simulink library "Project1_Library"  (R2017b)
settings: Solver=VariableStepAuto  StartTime=0.0  StopTime=10.0  RelTol=1e-3
settings Model: Creator=hattanbadyah  LastModifiedBy=hattanbadyah

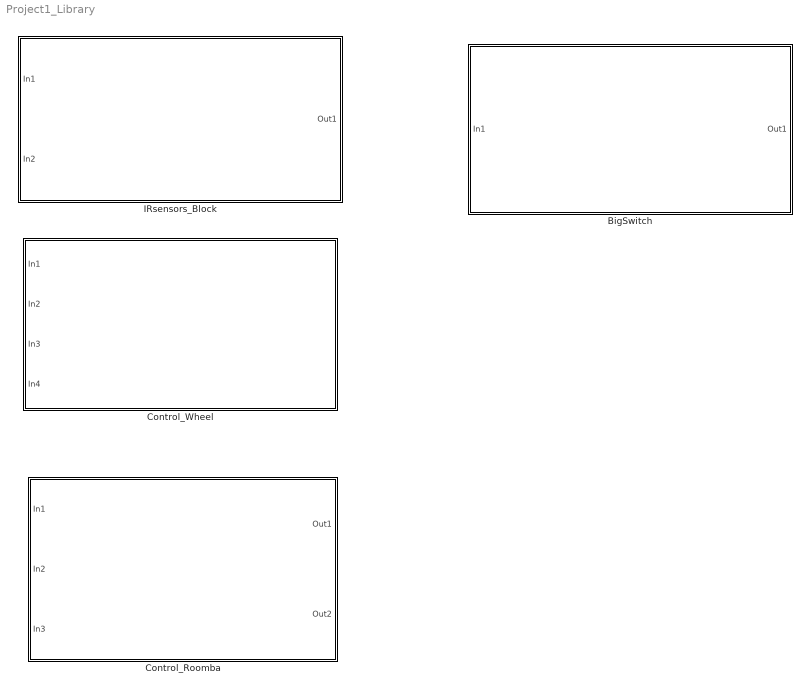
== system Project1_Library ==
  BigSwitch : Subsystem
      mask Help: Click on this link for more information:
      mask Display:
      | disp('BigSwitch');
      | port_label('output',1,'BigSwitch');
      | port_label('input', 1,'manual_switch');
  Control_Roomba : Subsystem
      mask help: This block contains the algorithm to control the Roomba and make it autonomus
      mask Display:
      | disp('Control_Roomba');
      | port_label('input', 1,'SonarSensor');
      | port_label('input', 2,'SonarRanges');
      | port_label('input', 3,'BigSwitch');
      | port_label('output',1,'LeftVel');
      | port_label('output',2,'RightVel');
  Control_Wheel : Subsystem
      mask Help: Click on this link for more information:
      mask Display:
      | disp('Control_Wheel');
      | port_label('input', 1,'LeftW');
      | port_label('input', 2,'RightW');
      | port_label('input', 3,'TurnWheel');
      | port_label('input', 4,'BigSwitch');
  IRsensors_Block : Subsystem
      mask Help: Click on this link for more information
      mask Display:
      | disp('IRsensors_Block');
      | port_label('input',1,'ReadSensor');
      | port_label('input', 2,'BigSwitch');
      | port_label('output', 1,'SensorsRead');

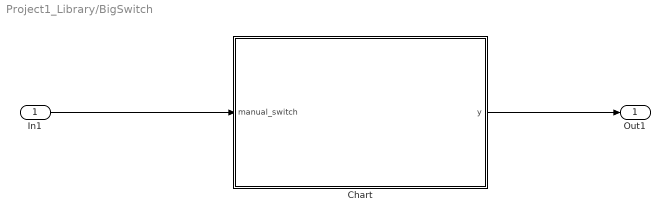
== system Project1_Library/BigSwitch ==
  In1 : Inport
  Chart : Stateflow chart  TreatAsAtomicUnit=on
  Out1 : Outport
  wires:
  In1/1 -> Chart/1(manual_switch)
  Chart/1(y) -> Out1/1

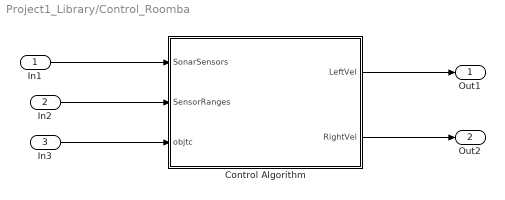
== system Project1_Library/Control_Roomba ==
  In1 : Inport
  In2 : Inport  Port=2
  In3 : Inport  Port=3
  Control Algorithm : Stateflow chart  TreatAsAtomicUnit=on  mask{v0=0.05}
      mask prompts: v0 "Wheel Angular Velocity"
  Out1 : Outport
  Out2 : Outport  Port=2
  wires:
  In1/1 -> Control Algorithm/1(SonarSensors)
  In2/1 -> Control Algorithm/2(SensorRanges)
  In3/1 -> Control Algorithm/3(objtc)
  Control Algorithm/1(LeftVel) -> Out1/1
  Control Algorithm/2(RightVel) -> Out2/1

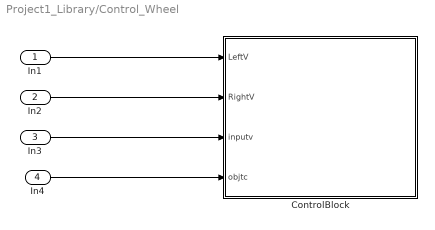
== system Project1_Library/Control_Wheel ==
  In1 : Inport
  In2 : Inport  Port=2
  In3 : Inport  Port=3
  In4 : Inport  Port=4
  ControlBlock : Stateflow chart  TreatAsAtomicUnit=on
  wires:
  In1/1 -> ControlBlock/1(LeftV)
  In2/1 -> ControlBlock/2(RightV)
  In3/1 -> ControlBlock/3(inputv)
  In4/1 -> ControlBlock/4(objtc)

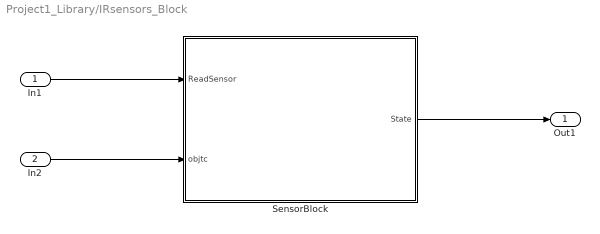
== system Project1_Library/IRsensors_Block ==
  In1 : Inport
  In2 : Inport  Port=2
  SensorBlock : Stateflow chart  TreatAsAtomicUnit=on
  Out1 : Outport
  wires:
  In1/1 -> SensorBlock/1(ReadSensor)
  In2/1 -> SensorBlock/2(objtc)
  SensorBlock/1(State) -> Out1/1

== stateflow chart Project1_Library/IRsensors_Block/SensorBlock ==
  state A
  state Start
    entry, during:
    coder.extrinsic('evalin')
    so=evalin('base','objWs');
    %status = 0
  state Sensor
    entry, during:
    coder.extrinsic('RangeStateRoomba');
    State=RangeStateRoomba(so);
    %status = 1;
  (default) -> A
  A -> Start : [objtc==1]
  Start -> Sensor : [ReadSensor==1]
  Sensor -> Start : [ReadSensor==0]
  data: ReadSensor input; so local; State output double size=6; objtc input

== stateflow chart Project1_Library/BigSwitch/Chart ==
  state A
    en,du:
    tcpInit;
  state Connect
    entry:
    y=1
  state Disconnect
    entry: coder.extrinsic('evalin');
    so=evalin('base','objWs');
    fclose(so);
  state Refresh1
    entry:
    y = y + 1
    if y==4
    y = 1
    end
  state Refresh
    entry:
    y = y + 1
  (default) -> A
  Disconnect -> A : [manual_switch==1]
  A -> Connect : [manual_switch==1]
  Refresh1 -> Connect [order 1] : [manual_switch==1]
  Connect -> Refresh : [manual_switch==1]
  Refresh1 -> Disconnect [order 2] : [manual_switch==0]
  Refresh -> Refresh1 : [manual_switch==1 ]
  data: manual_switch input; so local; y output
  function tcpInit:
    | function tcpInit
    | coder.extrinsic('tcpip');
    | coder.extrinsic('assignin');
    | persistent obj
    | if isempty(obj)
    |     obj=tcpip('10.0.0.1',9001);
    |     set(obj,'Terminator','LF')
    |     set(obj,'InputBufferSize',1000)
    |     set(obj, 'Timeout', 1)
    |     set(obj, 'ByteOrder','bigEndian');
    |     assignin('base','objWs',obj);
    |     
    | fopen(obj);
    |     % Start!
    | Start=[128];
    | fwrite(obj,Start);
    | pause(.1)
    | Mode=[132]
    | fwrite(obj,Mode);
    | pause(.1)
    | 
    | % %Print 'go' on display
    | fwrite(obj, [164, 71, 79, 32, 32]);
    | % make a sound
    | fwrite(obj, [140 1 3 60 20 72 20 84 40 ]); %RoombaInit Song
    | fwrite(obj, [140 2 1 60 20]); % BeepRoomba song
    | fwrite(obj, [140 3 3 84 20 72 30 60 40]); % PowerOffRoomba song
    | fwrite(obj, [141 1]); % play RoombaInit song
    | disp('Robot should display go on 7 segment LED panel and play song.')
    | pause(1);
    | end

== stateflow chart Project1_Library/Control_Wheel/ControlBlock ==
  state blank
  state Connect
    entry:
    coder.extrinsic('evalin');
    obj=evalin('base','objWs');
    %status= 0
  state Reset_Stop
    entry:
    coder.extrinsic('SetWheelVelRoomba')
    SetWheelVelRoomba(obj,0, 0)
    %status=2
  state Update
    entry,during:
    coder.extrinsic('SetWheelVelRoomba')
    SetWheelVelRoomba(obj,RightV, LeftV)
    %status=1
  state start
    entry,during:
    coder.extrinsic('SetWheelVelRoomba')
    SetWheelVelRoomba(obj,RightV, LeftV)
    %status=1
  (default) -> blank
  blank -> Connect : [objtc==2]
  Reset_Stop -> Connect [order 2] : after(30,sec)
  Connect -> start : [inputv==1]
  Update -> start : after(0.5,sec)
  start -> Reset_Stop [order 1] : [inputv==0]
  Reset_Stop -> start [order 1] : [inputv==1]
  start -> Update [order 2] : after(0.5,sec)
  data: LeftV input; RightV input; inputv input; objtc input; obj local

== stateflow chart Project1_Library/Control_Roomba/Control Algorithm ==
  state Begin
  state Control_Roomba
    en,du:
    coder.extrinsic('evalin');
    so=evalin('base','objWs');
    coder.extrinsic('PowerOffRoomba');
    coder.extrinsic('BatteryChargeReaderRoomba');
    coder.extrinsic('BeepRoomba');
    coder.extrinsic('BumpsWheelDropsSensorsRoomba');
    b_s= BumpsWheelDropsSensorsRoomba(so);
    coder.extrinsic('SeekDockRoomba');
    state Controling_Logic [parallel]
      en,du:
      RHS = [SonarSensors(4:6)] > SensorRanges(4:6);
      LHS = [SonarSensors(1:3)] > SensorRanges(1:3);
      MRS = [SonarSensors(5:6)] > SensorRanges(5:6);
      FRS = [SonarSensors(4:5)] > SensorRanges(4:5);
      FMS = [SonarSensors(3:4) ]> SensorRanges(3:4);
      FLS=[SonarSensors(2:3)]>SensorRanges(2:3);
      MLS=[SonarSensors(1:2)]>SensorRanges(1:2);
      RS1=[SonarSensors(6)]>SensorRanges(6);
      RS2=[SonarSensors(5)]>SensorRanges(5);
      RS3=[SonarSensors(4)]>SensorRanges(4);
      LS3=[SonarSensors(3)]>SensorRanges(3);
      LS2=[SonarSensors(2)]>SensorRanges(2);
      LS1=[SonarSensors(1)]>SensorRanges(1);
      R_bump=0;
      R_bump=b_s(1);
      L_bump=0;
      L_bump=b_s(2);
      F_bump=0;
      F_bump=b_s(3);
      WD_R=0;
      WD_R=b_s(4);
      WD_L=0;
      WD_L=b_s(5) ;
      settings: executionOrder=2
      state Start
      state Choose_None3
        en,du:
        RightVel=-v0;
        LeftVel=v0;
      state test_bump
        en,du:
        RightVel=-v0;
        LeftVel=-v0;
      state Choose_None
        en,du:
        RightVel= v0
        LeftVel= v0
      state Choose_None1
        en,du:
        RightVel= -v0
        LeftVel= v0
      state Front_S
        en,du:
        RightVel= -v0
        LeftVel= -v0
      state Choose_State
      state Choose_Between1
      state Choose_Between
      state Pick_LHS
        en,du:
        RightVel= -v0;
        LeftVel= -v0;
      state Pick_RHS
        en,du:
        RightVel= -v0;
        LeftVel= -v0;
      state Pick_RS3
        en,du:
        RightVel= v0;
        LeftVel= -v0 ;
      state Pick_RS2
        en,du:
        RightVel= v0;
        LeftVel= -v0;
      state Pick_MRS
        en,du:
        RightVel= v0;
        LeftVel= -v0;
      state Pick_FRS
        en,du:
        RightVel= v0;
        LeftVel= -v0;
      state Pick_RS1
        en,du:
        RightVel= v0;
        LeftVel= -v0;
      state Pick_LS3
        en,du:
        RightVel= -v0;
        LeftVel= v0;
      state Pick_MLS
        en,du:
        RightVel= -v0;
        LeftVel= v0;
      state Pick_FLS
        en,du:
        RightVel= -v0;
        LeftVel= v0;
      state Pick_LS1
        en,du:
        RightVel= -v0;
        LeftVel= v0;
      state Pick_LS2
        en,du:
        RightVel= -v0;
        LeftVel= v0;
      state Turnleft2
        en,du:
        RightVel= -v0;
        LeftVel= v0;
      state Turnleft1
        en,du:
        RightVel= v0;
        LeftVel= -v0;
      state wait2
      state Go_Straight
        en,du:
        RightVel = v0;
        LeftVel = v0;
      state Go_Straight1
        en,du:
        RightVel = v0;
        LeftVel = v0;
      state wait1
      (default) -> Start
      Start -> Choose_State : after(3,sec)
      test_bump -> Choose_None3
      Choose_None3 -> Choose_State : [R_bump<1&&L_bump<1&&F_bump<1&&WD_R<1&&WD_L<1]
      Choose_State -> test_bump [order 5] : [R_bump>0 | L_bump>0 | F_bump>0 | WD_R >0 | WD_L>0]
      Choose_None -> Choose_State
      Choose_State -> Choose_None [order 3] : [after(3,sec)]
      Choose_State -> Front_S [order 4] : [RS3>0&&LS3>0]
      Front_S -> Choose_None1
      Choose_None1 -> Choose_State : [RS3<1&&LS3<1]
      Choose_State -> Choose_Between1 [order 2] : [LHS(1)>0 | LHS(2)>0 | LHS(3) >0]
      Choose_State -> Choose_Between [order 1] : [RHS(1) >0 | RHS(2) > 0 | RHS(3)>0]
      Go_Straight -> Choose_State
      Go_Straight1 -> Choose_State
      Choose_Between1 -> Pick_LHS [order 1] : [LHS(1)>0&&LHS(2)>0&&LHS(3)>0]
      Choose_Between -> Pick_RHS [order 1] : [RHS(1)>0&&RHS(2)>0&&RHS(3)>0]
      Choose_Between -> Pick_RS3 [order 5] : [RS3>0]
      Choose_Between1 -> Pick_LS3 [order 6] : [LS3>0]
      Choose_Between1 -> Pick_LS2 [order 5] : [LS2>0]
      Choose_Between -> Pick_MRS [order 2] : [MRS(1)>0&&MRS(2)>0]
      Choose_Between -> Pick_RS2 [order 4] : [RS2>0]
      Choose_Between1 -> Pick_LS1 [order 4] : [LS1>0]
      Choose_Between -> Pick_FRS [order 6] : [FRS(1)>0&&FRS(2)]
      Choose_Between -> Pick_RS1 [order 3] : [RS1>0]
      Choose_Between1 -> Pick_MLS [order 2] : [MLS(1)>0&&MLS(2)>0]
      Choose_Between1 -> Pick_FLS [order 3] : [FLS(1)>0&&FLS(2)>0]
      Pick_LHS -> Turnleft2 : [after(3,sec)]
      Pick_RHS -> Turnleft1 : [after(3,sec)]
      Pick_RS3 -> Go_Straight : [RS3<1]
      Pick_RS2 -> Go_Straight : [RS2<1]
      Pick_RS1 -> Go_Straight : [RS1<1]
      Pick_MRS -> Go_Straight : [MRS(1)<1&&MRS(2)<1]
      Pick_FRS -> Go_Straight : [FRS(1)<1&&FRS(2)<1]
      Pick_MLS -> Go_Straight1 : [MLS(1)<1&&MLS(2)<1]
      Pick_LS1 -> Go_Straight1 : [LS1<1]
      Pick_LS2 -> Go_Straight1 : [LS2<1]
      Pick_LS3 -> Go_Straight1 : [LS3<1]
      Pick_FLS -> Go_Straight1 : [FLS(1)<1&&FLS(2)<1]
      Turnleft2 -> wait2 : [LHS(1)<1&&LHS(2)<1&&LHS(3)<1]
      wait2 -> Go_Straight1 : [after(10,sec)]
      Turnleft1 -> wait1 : [RHS(1)<1&&RHS(2)<1&&RHS(3)<1]
      wait1 -> Go_Straight : [after(10,sec)]
    state Parallel_State [parallel]
      settings: executionOrder=1
      state Monitor
        en,du:
        per= BatteryChargeReaderRoomba(so);
      state Stop
        en,du:
        BeepRoomba(so);
        BeepRoomba(so) ;
        PowerOffRoomba(so);
        coder.extrinsic('evalin');
        so=evalin('base','objWs');
        fclose(so);
      state Go_charge
        entry,du:
        SeekDockRoomba(so)
      (default) -> Monitor : {per=100}
      Go_charge -> Monitor : [per>20]
      Monitor -> Go_charge [order 2] : [per<=20]
      Stop -> Monitor : [per>15]
      Monitor -> Stop [order 1] : [per<=15]
  (default) -> Begin
  Begin -> Control_Roomba : [objtc==3]
  data: LeftVel output; RightVel output; SonarSensors input; SensorRanges input; v0 parameter; RS2 local; RHS local; RS3 local; FLS local; FRS local; FMS local; LS3 local; LS2 local; LS1 local; RS1 local; MLS local; LHS local; MRS local; objtc input; per local; so local; perc local; L_bump local; R_bump local; F_bump local; b_s local; WD_R local; WD_L local
